simulink library "uavsimBlockset_landinggear_onwheel"  (Simulink 8.0)
settings: Solver=ode45  StartTime=0.0  StopTime=10.0  RelTol=1e-3
libraries: uavsimblockset x4, aerolibutil x2
settings Model: Creator=mstolle  LastModifiedBy=j.bolting

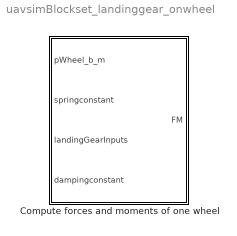
== system uavsimBlockset_landinggear_onwheel ==
  Compute forces and moments of one wheel : Subsystem

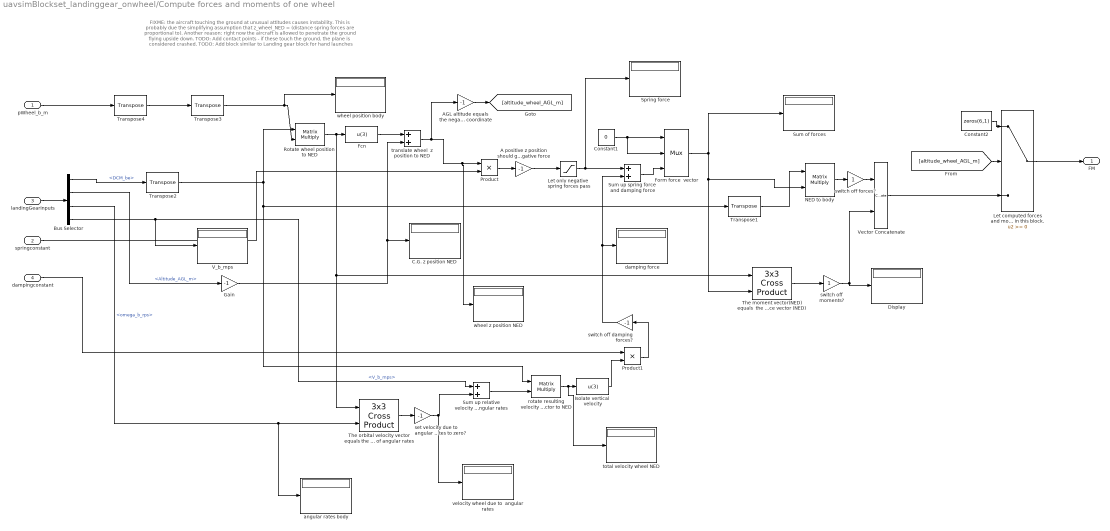
== system uavsimBlockset_landinggear_onwheel/Compute forces and moments of one wheel ==
  note: FIXME: the aircraft touching the ground at unusual attitudes causes instability. This is probably due the
      | simplifying assumption that z_wheel_NED = (distance spring forces are proportional to).
      | Another reason: right now the aircraft is allowed to penetrate the ground flying upside down.
      | TODO: Add contact points - if these touch the ground, the plane is considered crashed.
      | TODO: Add block similar to Landing gear block for hand launches
  pWheel_b_m : Inport
  springconstant : Inport  Port=2
  landingGearInputs : Inport  Port=3  OutDataTypeStr=Bus: LandinggearInput
  dampingconstant : Inport  Port=4
  A positive z position should generate  a negative force : Gain  Gain=-1
  AGL altitude equals the negative NED  z coordinate : Gain  Gain=-1
  Bus Selector : BusSelector  OutputSignals=DCM_be,Altitude_AGL_m,omega_b_rps,V_b_mps
  C.G. z position NED : Display
  Constant1 : Constant  Value=0
  Constant2 : Constant  Value=zeros(6,1)
  Display : Display
  Fcn : Fcn  Expr=u(3)
  Form force  vector : Mux  Inputs=3
  Gain : Gain  Gain=-1
  Isolate vertical  velocity : Fcn  Expr=u(3)
  Let computed forces and moments only pass if the wheel touches the ground. Thi s saves checking this condition multiple times in this block. : Switch
  Let only negative  spring forces pass : Saturate  UpperLimit=0  LowerLimit=-inf
  NED to body : Product  Multiplication=Matrix(*)
  Product : Product  RndMeth=Zero
  Product1 : Product  RndMeth=Zero
  Rotate wheel position  to NED : Product  Multiplication=Matrix(*)
  Spring force : Display
  Sum of forces : Display
  Sum up relative velocity of body frame and ground and velocity in the body frame  due to angular rates : Sum
  Sum up spring force  and damping force : Sum
  The moment vector(NED) equals  the cross product of the lever arm (NED) and the force vector (NED) : aerolibutil/3x3 Cross Product
  The orbital velocity vector equals the cross product of the radius vector (= position of the wheel in the body frame) and the vector of angular rates : aerolibutil/3x3 Cross Product
  Transpose{1..4} (4 alike) : uavsimblockset/Transpose  SystemSampleTime=-1
  V_b_mps : Display
  Vector Concatenate : Concatenate
  angular rates body : Display
  damping force : Display
  rotate resulting velocity vector to NED : Product  Multiplication=Matrix(*)
  set velocity due to angular rates to zero? : Gain  Gain=-1
  switch off damping forces? : Gain  Gain=-1
  switch off forces? : Gain
  switch off moments? : Gain
  total velocity wheel NED : Display
  translate wheel  z position to NED : Sum
  velocity wheel due to  angular rates : Display
  wheel position body : Display
  "wheel z position NED " : Display
  FM : Outport
  wires:
  Transpose3/1 -> wheel position body/1, Rotate wheel position  to NED/2
  Let computed forces and moments only pass if the wheel touches the ground. Thi s saves checking this condition multiple times in this block./1 -> FM/1
  Vector Concatenate/1 -> Let computed forces and moments only pass if the wheel touches the ground. Thi s saves checking this condition multiple times in this block./3
  Constant2/1 -> Let computed forces and moments only pass if the wheel touches the ground. Thi s saves checking this condition multiple times in this block./1
  [altitude_wheel_AGL_m] -> Let computed forces and moments only pass if the wheel touches the ground. Thi s saves checking this condition multiple times in this block./2
  AGL altitude equals the negative NED  z coordinate/1 -> [altitude_wheel_AGL_m]
  set velocity due to angular rates to zero?/1 -> velocity wheel due to  angular rates/1, Sum up relative velocity of body frame and ground and velocity in the body frame  due to angular rates/2
  switch off damping forces?/1 -> Sum up spring force  and damping force/2, damping force/1
  switch off forces?/1 -> Vector Concatenate/1
  switch off moments?/1 -> Vector Concatenate/2, Display/1
  The moment vector(NED) equals  the cross product of the lever arm (NED) and the force vector (NED)/1 -> switch off moments?/1
  Transpose1/1 -> NED to body/1
  NED to body/1 -> switch off forces?/1
  Transpose4/1 -> Transpose3/1
  pWheel_b_m/1 -> Transpose4/1
  Bus Selector/1 -> Transpose2/1  "<DCM_be>"
  springconstant/1 -> Product/2
  Bus Selector/2 -> Gain/1  "<Altitude_AGL_m>"
  translate wheel  z position to NED/1 -> Product/1, "wheel z position NED "/1, AGL altitude equals the negative NED  z coordinate/1
  Fcn/1 -> translate wheel  z position to NED/1
  Gain/1 -> C.G. z position NED/1, translate wheel  z position to NED/2
  Constant1/1 -> Form force  vector/2, Form force  vector/1
  Product/1 -> A positive z position should generate  a negative force/1
  A positive z position should generate  a negative force/1 -> Let only negative  spring forces pass/1
  Form force  vector/1 -> NED to body/2, The moment vector(NED) equals  the cross product of the lever arm (NED) and the force vector (NED)/2, Sum of forces/1
  Sum up spring force  and damping force/1 -> Form force  vector/3
  Let only negative  spring forces pass/1 -> Sum up spring force  and damping force/1, Spring force/1
  landingGearInputs/1 -> Bus Selector/1
  Transpose2/1 -> Rotate wheel position  to NED/1, rotate resulting velocity vector to NED/1, Transpose1/1
  Rotate wheel position  to NED/1 -> The orbital velocity vector equals the cross product of the radius vector (= position of the wheel in the body frame) and the vector of angular rates/1, The moment vector(NED) equals  the cross product of the lever arm (NED) and the force vector (NED)/1, Fcn/1
  Bus Selector/3 -> angular rates body/1, The orbital velocity vector equals the cross product of the radius vector (= position of the wheel in the body frame) and the vector of angular rates/2  "<omega_b_rps>"
  The orbital velocity vector equals the cross product of the radius vector (= position of the wheel in the body frame) and the vector of angular rates/1 -> set velocity due to angular rates to zero?/1
  Bus Selector/4 -> Sum up relative velocity of body frame and ground and velocity in the body frame  due to angular rates/1, V_b_mps/1  "<V_b_mps>"
  dampingconstant/1 -> Product1/1
  Product1/1 -> switch off damping forces?/1
  Sum up relative velocity of body frame and ground and velocity in the body frame  due to angular rates/1 -> rotate resulting velocity vector to NED/2
  rotate resulting velocity vector to NED/1 -> total velocity wheel NED/1, Isolate vertical  velocity/1
  Isolate vertical  velocity/1 -> Product1/2
